simulink model "integratorbloack_externalVariable"  (R2024b)
settings: Solver=VariableStepAuto  StartTime=0.0  StopTime=10.0  RelTol=1e-3
values from neighbouring files (symbols this model uses):
  ui = input("enter number: ")    [integratorbloack_externalVariable_mfile.m]
settings Model: Creator=admin  LastModifiedBy=admin

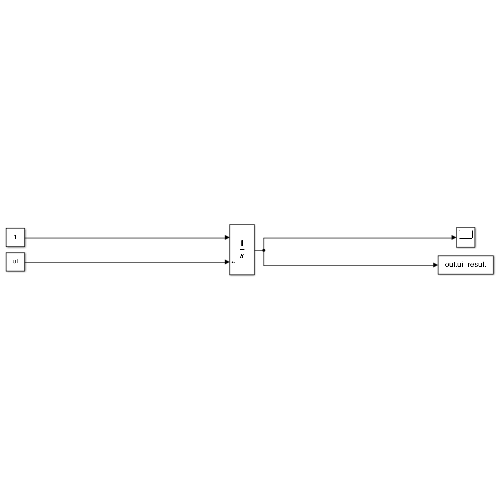
[thumbnail: Simulink's stored preview of the top-level diagram]
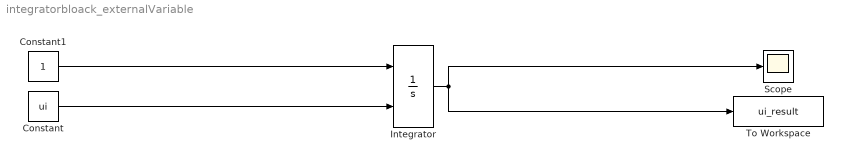
== system integratorbloack_externalVariable ==
  Constant : Constant  Value=ui
  Constant1 : Constant
  Integrator : Integrator  InitialConditionSource=external  InitialCondition=5
  Scope : Scope
  To Workspace : ToWorkspace  VariableName=ui_result  SaveFormat=Timeseries  SampleTime=-1
  wires:
  Constant/1 -> Integrator/2
  Integrator/1 -> Scope/1, To Workspace/1
  Constant1/1 -> Integrator/1
